simulink model "questao2"  (Simulink 6.0)
settings: Solver=ode45  StartTime=0.0  StopTime=1000.0  RelTol=1e-3
settings Model: Creator=usuario  LastModifiedBy=Thales Ruano
settings OptimizationCC: InlineInvariantSignals=off
settings DebuggingCC: SignalResolutionControl=UseLocalSettings
settings GRTTargetCC: TargetFcnLib=ansi_tfl_table_tmw.mat

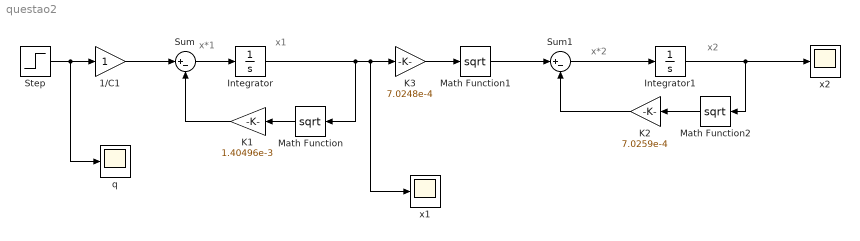
== system questao2 ==
  note: x*1
  note: x1
  note: x*2
  note: x2
  1/C1 : Gain
  Integrator : Integrator  InitialCondition=5
  Integrator1 : Integrator  InitialCondition=2
  K1 : Gain  Orientation=left  Gain=1.40496e-3
  K2 : Gain  Orientation=left  Gain=7.0259e-4
  K3 : Gain  Gain=7.0248e-4
  Math Function : Math  Orientation=left  Operator=sqrt  SaturateOnIntegerOverflow=on
  Math Function1 : Math  Operator=sqrt  SaturateOnIntegerOverflow=on
  Math Function2 : Math  Orientation=left  Operator=sqrt  SaturateOnIntegerOverflow=on
  Step : Step  Time=0  After=0.5e-3  SampleTime=0
  Sum : Sum  Inputs=|+-
  Sum1 : Sum  Inputs=|+-
  q : Scope
      settings: SaveName=ScopeData2
  x1 : Scope
  x2 : Scope
  wires:
  Step/1 -> 1/C1/1, q/1
  1/C1/1 -> Sum/1
  Sum/1 -> Integrator/1
  K1/1 -> Sum/2
  Math Function/1 -> K1/1
  Integrator/1 -> Math Function/1, K3/1, x1/1
  K3/1 -> Math Function1/1
  Math Function1/1 -> Sum1/1
  K2/1 -> Sum1/2
  Math Function2/1 -> K2/1
  Sum1/1 -> Integrator1/1
  Integrator1/1 -> Math Function2/1, x2/1
